simulink subsystem "gq_SubSystem"  (R2020b)
settings: Solver=VariableStepAuto  StartTime=0.0  StopTime=10.0  RelTol=1e-3
values from neighbouring files (symbols this model uses):
  g = 9.81    [balrob_params.m]
  g1q = 0    [Electromechanical.m]
  l = body.zb    [Electromechanical.m]
  mb = body.m    [Electromechanical.m]
  mrot = mot.rot.m    [Electromechanical.m]
  Ts = 1e-2    (= 0.01)    [balrob_params.m]
  zbrot = mot.rot.zb    [Electromechanical.m]
settings Model: Creator=umberto  LastModifiedBy=umberto

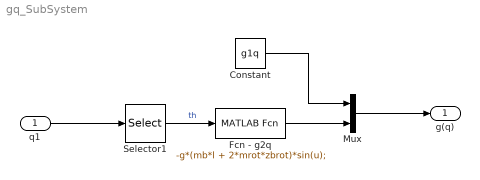
== system gq_SubSystem ==
  q1 : Inport
  Constant : Constant  Value=g1q  SampleTime=Ts
  Fcn - g2q : MATLABFcn  MATLABFcn=-g*(mb*l + 2*mrot*zbrot)*sin(u);
  Mux : Mux  Inputs=2
  Selector1 : Selector  InputPortWidth=2  IndexOptions=Index vector (dialog)  Indices=[2]  OutputSizes=1
  g(q) : Outport
  wires:
  Selector1/1 -> Fcn - g2q/1  "th"
  q1/1 -> Selector1/1
  Fcn - g2q/1 -> Mux/2
  Constant/1 -> Mux/1
  Mux/1 -> g(q)/1
